simulink library "manageILCTriggers_ul"  (R2018a)
settings: Solver=VariableStepAuto  StartTime=0.0  StopTime=10.0  RelTol=1e-3
settings Model: Creator=mitch  LastModifiedBy=M.Cobb

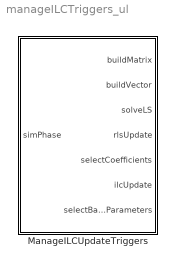
== system manageILCTriggers_ul ==
  ManageILCUpdateTriggers : Subsystem

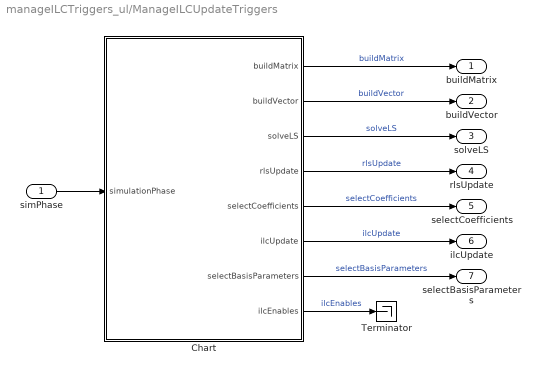
== system manageILCTriggers_ul/ManageILCUpdateTriggers ==
  simPhase : Inport
  Chart : Stateflow chart  TreatAsAtomicUnit=on
  Terminator : Terminator
  buildMatrix : Outport  OutDataTypeStr=boolean
  buildVector : Outport  Port=2  OutDataTypeStr=boolean
  solveLS : Outport  Port=3  OutDataTypeStr=boolean
  rlsUpdate : Outport  Port=4  OutDataTypeStr=boolean
  selectCoefficients : Outport  Port=5  OutDataTypeStr=boolean
  ilcUpdate : Outport  Port=6  OutDataTypeStr=boolean
  selectBasisParameters : Outport  Port=7  OutDataTypeStr=boolean
  wires:
  Chart/8(ilcEnables) -> Terminator/1  "ilcEnables"
  simPhase/1 -> Chart/1(simulationPhase)
  Chart/7(selectBasisParameters) -> selectBasisParameters/1  "selectBasisParameters"
  Chart/6(ilcUpdate) -> ilcUpdate/1  "ilcUpdate"
  Chart/5(selectCoefficients) -> selectCoefficients/1  "selectCoefficients"
  Chart/4(rlsUpdate) -> rlsUpdate/1  "rlsUpdate"
  Chart/3(solveLS) -> solveLS/1  "solveLS"
  Chart/2(buildVector) -> buildVector/1  "buildVector"
  Chart/1(buildMatrix) -> buildMatrix/1  "buildMatrix"

== stateflow chart manageILCTriggers_ul/ManageILCUpdateTriggers/Chart ==
  state SETTLING
    buildMatrix = false;
    buildVector = false;
    solveLS = false;
    rlsUpdate = false;
    selectCoefficients = false;
    ilcUpdate = false;
    selectBasisParameters = false;
  state STARTBUILDINGMATRIX
    buildMatrix = true;
  state STARTBUILDINGVECTOR
    buildVector  = true;
  state STARTOPTIMIZATION
    buildMatrix = false;
    buildVector = true;
    solveLS = true;
    rlsUpdate = true;
    selectCoefficients = true;
    selectBasisParameters = true;
  state FREERUNOPTIMIZATION
    buildVector = false;
    solveLS = false;
    ilcUpdate = true;
  (default) -> SETTLING
  SETTLING -> STARTBUILDINGMATRIX : [simulationPhase == simulationPhase_enum.INITIALIZATION]
  STARTBUILDINGMATRIX -> STARTBUILDINGVECTOR : after(1,tick)
  STARTBUILDINGVECTOR -> STARTOPTIMIZATION : [simulationPhase == simulationPhase_enum.OPTIMIZATION]
  STARTOPTIMIZATION -> FREERUNOPTIMIZATION : after(1,tick)
  data: buildMatrix output boolean; buildVector output boolean; solveLS output boolean; rlsUpdate output boolean; selectCoefficients output boolean; ilcUpdate output boolean; selectBasisParameters output boolean; simulationPhase input Enum: simulationPhase_enum; ilcEnables output Enum: ilcEnables_enum
